simulink subsystem "station1"  (R2024b)
settings: Solver=VariableStepAuto  StartTime=0.0  StopTime=10.0  RelTol=1e-3
undefined symbols (not defined in the file): DiscIntNeverNeededParam, DPL1ph, h, Half, R3, ResistanceM, Rt4, simetran, Ts, Zm
libraries: fl_lib x215, ee_lib x97, nesl_utility x43, spsThreePhaseHarmonicFilterLib x21, simulink x7, spsThreePhaseSeriesRLCLoadLib x7, spsThreePhaseBreakerLib x7
(part 1 of 6)
settings Model: Creator=Kyle  LastModifiedBy=CD8435

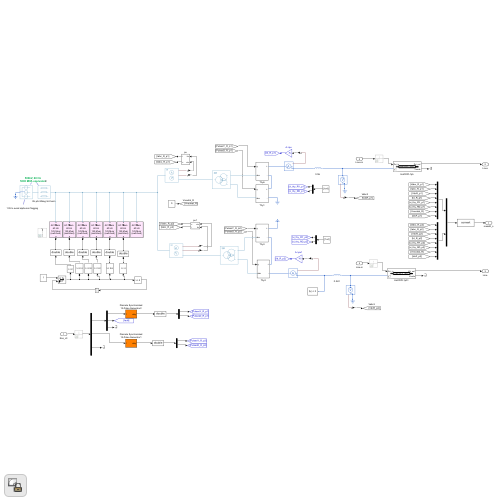
[thumbnail: Simulink's stored preview of the top-level diagram]
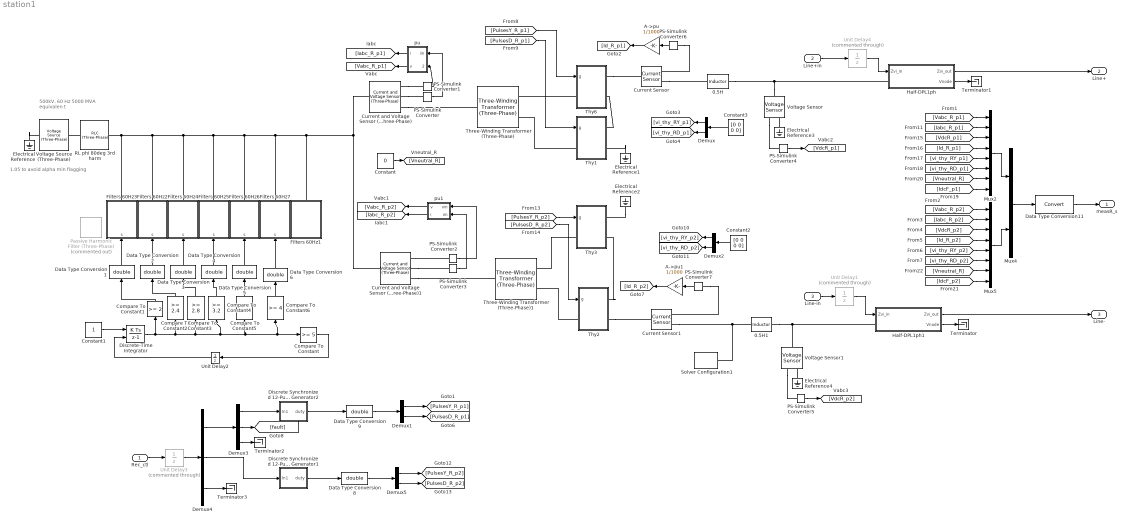
== system station1 ==
  note: 1.05 to avoid alpha min flagging
  note: 500kV, 60 Hz
      | 5000 MVA equivalen t
  Rec_ctl : Inport
  Line+in : Inport  Port=2
  Line-in : Inport  Port=3
  0.5H : ee_lib/Passive/Inductor  l=0.5 H  enable_L_tol=ee.enum.toleranceApplication.none  L_tol=20  tol_distribution=ee.enum.toleranceDistribution.uniform  nSigma=4  r=1 Ohm  g=1e-9 1/Ohm  enable_operating_limits=ee.enum.enable.no  operating_limit_action=ee.enum.passive.reportOpLim.warn  max_working_current=1 A  power_rating=1 W  fault_action=simscape.enum.assert.action.none  t_fault=1 s  i_L_specify=off  i_L_priority=High  i_L=0 A  i_L_nominal_specify=off  i_L_nominal_value=1  i_L_nominal_unit=A
  0.5H1 : ee_lib/Passive/Inductor  l=0.5 H  enable_L_tol=ee.enum.toleranceApplication.none  L_tol=20  tol_distribution=ee.enum.toleranceDistribution.uniform  nSigma=4  r=1 Ohm  g=1e-9 1/Ohm  enable_operating_limits=ee.enum.enable.no  operating_limit_action=ee.enum.passive.reportOpLim.warn  max_working_current=1 A  power_rating=1 W  fault_action=simscape.enum.assert.action.none  t_fault=1 s  i_L_specify=off  i_L_priority=High  i_L=0 A  i_L_nominal_specify=off  i_L_nominal_value=1  i_L_nominal_unit=A
  A->pu : Gain  Gain=1/1000  SaturateOnIntegerOverflow=on  OutDataTypeStr=Inherit: Same as input  ParamDataTypeStr=Inherit: Same as input
  A->pu1 : Gain  Gain=1/1000  SaturateOnIntegerOverflow=on  OutDataTypeStr=Inherit: Same as input  ParamDataTypeStr=Inherit: Same as input
  Compare To Constant : simulink/Logic and Bit Operations/Compare To Constant  relop=>=  const=5  OutDataTypeStr=uint8  ZeroCross=off
  Compare To Constant1 : simulink/Logic and Bit Operations/Compare To Constant  relop=>=  const=2  OutDataTypeStr=uint8  ZeroCross=off
  Compare To Constant2 : simulink/Logic and Bit Operations/Compare To Constant  relop=>=  const=2.4  OutDataTypeStr=uint8  ZeroCross=off
  Compare To Constant3 : simulink/Logic and Bit Operations/Compare To Constant  relop=>=  const=2.8  OutDataTypeStr=uint8  ZeroCross=off
  Compare To Constant4 : simulink/Logic and Bit Operations/Compare To Constant  relop=>=  const=3.2  OutDataTypeStr=uint8  ZeroCross=off
  Compare To Constant5 : simulink/Logic and Bit Operations/Compare To Constant  relop=>=  const=3.6  OutDataTypeStr=uint8  ZeroCross=off
  Compare To Constant6 : simulink/Logic and Bit Operations/Compare To Constant  relop=>=  const=4  OutDataTypeStr=uint8  ZeroCross=off
  Constant : Constant  Value=0
  Constant1 : Constant
  Constant2 : Constant  Value=[0 0 0 0]
  Constant3 : Constant  Value=[0 0 0 0]
  Current Sensor : fl_lib/Electrical/Electrical Sensors/Current Sensor
  Current Sensor1 : fl_lib/Electrical/Electrical Sensors/Current Sensor
  Current and Voltage Sensor (Three-Phase) : ee_lib/Sensors & Transducers/Current and Voltage Sensor (Three-Phase)  vMeasurementType=ee.enum.vmeasurement.lg  outputUnit=ee.enum.unit.si  SRated=100e6 A*V  VRated=24e3 V  I_specify=off  I_priority=None  I=[0, 0, 0] A  I_nominal_specify=off  I_nominal_value=1  I_nominal_unit=A  V_specify=off  V_priority=None  V=[0, 0, 0] V  V_nominal_specify=off  V_nominal_value=1  V_nominal_unit=V
      settings: InternalSimscapePortConfiguration="{\"Bottom\":[],\"Left\":[{\"id\":\"N1\",\"label\":\"~1\",\"type\":\"foundation.electrical.three_phase\"}],\"Right\":[{\"id\":\"V_output\",\"label\":\"V\",\"type\":\"output\"},{\"id\":\"I_output\",\"label\":\"I\",\"type\":\"output\"},{\"id\":\"N2\",\"label\":\"~2\",\"type\":\"foundation.electrical.three_phase\"}],\"Top\":[]}"
  Current and Voltage Sensor (Three-Phase)1 : ee_lib/Sensors & Transducers/Current and Voltage Sensor (Three-Phase)  vMeasurementType=ee.enum.vmeasurement.lg  outputUnit=ee.enum.unit.si  SRated=100e6 A*V  VRated=24e3 V  I_specify=off  I_priority=None  I=[0, 0, 0] A  I_nominal_specify=off  I_nominal_value=1  I_nominal_unit=A  V_specify=off  V_priority=None  V=[0, 0, 0] V  V_nominal_specify=off  V_nominal_value=1  V_nominal_unit=V
      settings: InternalSimscapePortConfiguration="{\"Bottom\":[],\"Left\":[{\"id\":\"N1\",\"label\":\"~1\",\"type\":\"foundation.electrical.three_phase\"}],\"Right\":[{\"id\":\"V_output\",\"label\":\"V\",\"type\":\"output\"},{\"id\":\"I_output\",\"label\":\"I\",\"type\":\"output\"},{\"id\":\"N2\",\"label\":\"~2\",\"type\":\"foundation.electrical.three_phase\"}],\"Top\":[]}"
  Data Type Conversion{1..6,8..9} (8 alike) : DataTypeConversion  OutDataTypeStr=double  SaturateOnIntegerOverflow=off  RndMeth=Floor
  Data Type Conversion11 : DataTypeConversion  SaturateOnIntegerOverflow=off  RndMeth=Floor
  Demux : Demux  Outputs=2
  Demux1 : Demux  Outputs=[6 6]
  Demux2 : Demux  Outputs=2
  Demux3 : Demux  Outputs=[6 1 1]
  Demux4 : Demux  Outputs=[8 6 1]
  Demux5 : Demux  Outputs=[6 6]
  Discrete Synchronized 12-Pulse Generator1 : Subsystem
  Discrete Synchronized 12-Pulse Generator2 : Subsystem
  Discrete-Time Integrator : DiscreteIntegrator  ExternalReset=rising  SampleTime=Ts  ICPrevOutput=DiscIntNeverNeededParam  ICPrevScaledInput=DiscIntNeverNeededParam
  Electrical Reference{,1..4} (5 alike) : fl_lib/Electrical/Electrical Elements/Electrical Reference
  Filters 60Hz1 : Subsystem
      mask Display: disp('AC filters \n60 Hz\n125 Mvar\n(switched)')
  Filters 60Hz2 : Subsystem
      mask Display: disp('AC filters \n60 Hz\n125 Mvar\n(switched)')
  Filters 60Hz3 : Subsystem
      mask Display: disp('AC filters \n60 Hz\n125 Mvar\n(switched)')
  Filters 60Hz4 : Subsystem
      mask Display: disp('AC filters \n60 Hz\n125 Mvar\n(switched)')
  Filters 60Hz5 : Subsystem
      mask Display: disp('AC filters \n60 Hz\n125 Mvar\n(switched)')
  Filters 60Hz6 : Subsystem
      mask Display: disp('AC filters \n60 Hz\n125 Mvar\n(switched)')
  Filters 60Hz7 : Subsystem
      mask Display: disp('AC filters \n60 Hz\n125 Mvar\n(switched)')
  Half-DPL1ph : Subsystem  AncestorBlock=simetran/Half-DPL1ph  mask(Simscape 1-phase Distributed Parameters Line){Phases=1, Frequency=60, Resistance=0.015, Inductance=0.792e-3, Capacitance=14.4e-9, Length=300, Ts=Ts, cd=on}
      mask prompts: Phases "Number of phases N"; Frequency "Frequency used for R L C specification (Hz)"; Resistance "Resistance per unit length (Ohms/km)   [N*N matrix] or [R1 R0 R0m]"; Inductance "Inductance per unit length (H/km) [N*N matrix ] or [L1 L0 L0m]"; Capacitance "Capacitance per unit length (F/km) [N*N matrix] or [C1 C0 C0m]"; Length "Line length (km)"; Ts "Sample time (s)"; cd "Compensate for explicit external Unit Delay of propagation"
      mask help:
      | Implements a single-phase distributed parameter line (DPL) model.
      |
      | This DPL model allows the decoupling of computational tasks at each line ends.
      mask init:
      | % Get current block
      | currentBlock = gcb;
      | 
      | % Get electric variables
      | [Zm,R,v,Ti,to,Rt4,h,Zimp,Zmat,Yphase,ResistanceM] = ssc_dpl_cb(gcb,'variable_mask_maskinitialization', Phases, Frequency, Resistance, Inductance, Capacitance, Length);
      | % nphase=Phases;
      | % [Zm,R,v,Ti]=powericon('Distributed Parameter Line Model',nphase,Frequency,Resistance,Inductance,Capacitance);
      | %         %[Zmxx,Rmxx,Smodexx,Tixx] = blmodlin(nphase,Frequency,Resistance,Inductance,Capacitance);
      | %         %warning(w);
      | % 
      | % 
      | %         to = Length ./ v;
      | %         Rt4 = R * Length / 4;
      | %         h = (Zm - Rt4) ./ (Zm + Rt4);
      | %         Zimp = Zm + Rt4;
      | % 
      | %         % Calculate Zmat
      | %         Zmat = zeros(nphase);
      | %         for t = 1 : nphase
      | %             Zmat(t,t) = Zimp(t);
      | %         end
      | % 
      | %         % Calculate Y phase
      | %         Yphase=Ti*inv(Zmat)*(Ti');
      | % 
      | %         % Calculate R_x_0
      | %         ResistanceM = zeros(nphase);
      | %         for t = 1 : nphase
      | %             ResistanceM(t,t) = 1/(sum(Yphase(t,1:nphase)));
      | %         end
      | % 
      | %         % Calculate R_m_n
      | %         for t = 1 : nphase
      | %             for u = t+1: nphase
      | %                 ResistanceM(t,u) = -1/(Yphase(u,t));
      | %             end
      | %         end
      | V1_init=[0 zeros(1,Phases); 0.1 zeros(1,Phases)];
      | delay=floor(to/Ts);
      | if cd==1
      |     delay=delay-1;
      | end
      | if delay<1
      |     error('Line delay is less than 1 time step');
      | end
      | remd=rem(to,Ts)/Ts;
      mask TypeOptions Phases: 1 | 2 | 3 | 4 | 5 | 6 | 8 | 9 | 10 | 12
      mask Display:
      | plot(0,0,100,100,[20,20,80,80,90,80,80,20,20,10],[50,40,40,50,50,50,61,61,50,50])
      | disp('half-DPL 1ph)')
      | %disp(mess)
  Half-DPL1ph1 : Subsystem  AncestorBlock=simetran/Half-DPL1ph  mask(Simscape 1-phase Distributed Parameters Line){Phases=1, Frequency=60, Resistance=0.015, Inductance=0.792e-3, Capacitance=14.4e-9, Length=300, Ts=Ts, cd=on}
      mask prompts: Phases "Number of phases N"; Frequency "Frequency used for R L C specification (Hz)"; Resistance "Resistance per unit length (Ohms/km)   [N*N matrix] or [R1 R0 R0m]"; Inductance "Inductance per unit length (H/km) [N*N matrix ] or [L1 L0 L0m]"; Capacitance "Capacitance per unit length (F/km) [N*N matrix] or [C1 C0 C0m]"; Length "Line length (km)"; Ts "Sample time (s)"; cd "Compensate for explicit external Unit Delay of propagation"
      mask help:
      | Implements a single-phase distributed parameter line (DPL) model.
      |
      | This DPL model allows the decoupling of computational tasks at each line ends.
      mask init: same as station1/Half-DPL1ph
      mask TypeOptions Phases: 1 | 2 | 3 | 4 | 5 | 6 | 8 | 9 | 10 | 12
      mask Display:
      | plot(0,0,100,100,[20,20,80,80,90,80,80,20,20,10],[50,40,40,50,50,50,61,61,50,50])
      | disp('half-DPL 1ph)')
      | %disp(mess)
  Mux2 : Mux  Inputs=[3 3 1 1 2 2 1 1]
  Mux4 : Mux  Inputs=[14 14 ]
  Mux5 : Mux  Inputs=[3 3 1 1 2 2 1 1]
  PS-Simulink Converter{,1..7} (8 alike) : nesl_utility/PS-Simulink Converter  PhysicalDomain=network_engine_domain  SubClassName=ps_output  LeftPortType=input  RightPortType=output  PseudoPeriodic=off  Frequencies=[]  VectorFormat=inherit  Unit=inherit  AffineConversion=off
  Passive Harmonic Filter (Three-Phase) : ee_lib/Passive/Passive Harmonic Filter (Three-Phase)  Commented=on  QRated=100e6 A*V  VRated=4160 V  FRated=60 Hz  qfactor=10  type_option=ee.enum.filtertype.BPsingle  connection_option=ee.enum.filterconnection.delta  ftuned=5 * 60 Hz  ftuned1=7 * 60 Hz  ftuned2=11 * 60 Hz  I_specify=off  I_priority=None  I=[0, 0, 0] A  I_nominal_specify=off  I_nominal_value=1  I_nominal_unit=A  V_specify=off  V_priority=None  V=[0, 0, 0] V  V_nominal_specify=off  V_nominal_value=1  V_nominal_unit=V
      settings: InternalSimscapePortConfiguration="{\"Bottom\":[],\"Left\":[{\"id\":\"N\",\"label\":\"~\",\"type\":\"foundation.electrical.three_phase\"}],\"Right\":[],\"Top\":[]}"
  RL phi 80deg 3rd harm : ee_lib/Passive/RLC Assemblies/RLC (Three-Phase)  port_option=ee.enum.threePhasePort.composite  component_structure=ee.enum.rlc.structure.ParallelRL  R=26.07 Ohm  L=48.86e-3 H  C=1e-6 F  R_parasitic=0 Ohm  G_parasitic=0 1/Ohm  IL_specify=off  IL_priority=High  IL=[0, 0, 0] A  IL_nominal_specify=off  IL_nominal_value=1  IL_nominal_unit=A  VC_specify=off  VC_priority=High  VC=[0, 0, 0] V  VC_nominal_specify=off  VC_nominal_value=1  VC_nominal_unit=V
      settings: InternalSimscapePortConfiguration="{\"Bottom\":[],\"Left\":[{\"id\":\"N1\",\"label\":\"~1\",\"type\":\"foundation.electrical.three_phase\"}],\"Right\":[{\"id\":\"N2\",\"label\":\"~2\",\"type\":\"foundation.electrical.three_phase\"}],\"Top\":[]}"
  Solver Configuration1 : nesl_utility/Solver Configuration  PhysicalDomain=network_engine_domain  SubClassName=solver  LeftPortType=input  RightPortType=generic  Tones=[]  Harmonics=[]  SimulateNoise=off  Profile=off  UseLocalSampling=off  EnableSwitchedLinearOptims=on  FrequencyDomain=off  UseCCode=off  RelTol=0.001  AbsTol=1e-06  MinStep=1e-09  ToWorkspace=off  RevertToSquareIcSolve=off  NumHomotopyIterations=100  PhasorMode=off  PhasorModeNumHarmonics=1  ConsistencySolver=NEWTON_FTOL  IndexReductionMethod=DerivativeReplacement  DoDC=off  ResidualTolerance=0.01  ConsistencyTolSource=GLOBAL  ConsistencyAbsTol=0.001  ConsistencyRelTol=0.001  ConsistencyTolFactor=0.001  UseLocalSolver=on  LocalSolverChoice=NE_BACKWARD_EULER_ADVANCER  ResolveIndetEquations=off  FunctionEvalNumThread=1  LocalSolverSampleTime=Ts  DoFixedCost=on  MaxNonlinIter=1  MaxModeIter=2  ComputeImpulses=off  ImpulseIterations=2  LinearAlgebra=Sparse  LinearAlgebraNumThread=0  EquationFormulation=NE_TIME_EF  DelaysMemoryBudget=1024  AutomaticFiltering=off  FilteringTimeConstant=0.001  PartitionStorageMethod=AS_NEEDED  PartitionMemoryBudget=1024  PartitionMethod=ROBUST  MultibodyUseLocalSolver=off  MultibodyLocalSolverChoice=ODE1  MultibodyLocalSolverSampleTime=0.001
  Terminator{,1..3} (4 alike) : Terminator
  Three-Winding Transformer (Three-Phase) : ee_lib/Passive/Transformers/Three-Winding Transformer (Three-Phase)  SRated=1200e6 A*V  FRated=60 Hz  Winding1Connection=ee.enum.windingconnection.Yg  VRated1=500e3*0.9 V  Winding2Connection=ee.enum.windingconnection.Y  VRated2=200e3 V  Winding3Connection=ee.enum.windingconnection.delta1  VRated3=200e3 V  CoreType=ee.enum.coretype.threelimb  pu_Rw1=0.0025  pu_Rw2=0.0025  pu_Rw3=0.0025  leakage_reactance_option=ee.enum.transformer_leakage.include  pu_Xl1=0.001  pu_Xl2=0.24  pu_Xl3=0.24  magnetizing_resistance_option=ee.enum.transformer_magnetizingResistance.include  pu_Rm=500  magnetizing_reactance_option=ee.enum.transformer_magnetizingReactance.exclude  saturation_option=ee.enum.transformer_saturation.exclude  pu_Xm=500  current_data=[0, .002, 1, 2]  magnetic_flux_data=[0, 1.2, 1.5, 1.51]  pu_X0=0.5  i1_specify=off  i1_priority=None  i1=[0, 0, 0] A  i1_nominal_specify=off  i1_nominal_value=1  i1_nominal_unit=A  i2_specify=off  i2_priority=None  i2=[0, 0, 0] A  i2_nominal_specify=off  i2_nominal_value=1  i2_nominal_unit=A  i3_specify=off  i3_priority=None  i3=[0, 0, 0] A  i3_nominal_specify=off  i3_nominal_value=1  i3_nominal_unit=A  phi_specify=off  phi_priority=None  phi=[0, 0, 0]  phi_nominal_specify=off  phi_nominal_value=1  phi_nominal_unit=1  power_dissipated_specify=off  power_dissipated_priority=None  power_dissipated=0 W  power_dissipated_nominal_specify=off  power_dissipated_nominal_value=1  power_dissipated_nominal_unit=W
      settings: InternalSimscapePortConfiguration="{\"Bottom\":[],\"Left\":[{\"id\":\"N1\",\"label\":\"~1\",\"type\":\"foundation.electrical.three_phase\"}],\"Right\":[{\"id\":\"N2\",\"label\":\"~2\",\"type\":\"foundation.electrical.three_phase\"},{\"id\":\"N3\",\"label\":\"~3\",\"type\":\"foundation.electrical.three_phase\"}],\"Top\":[]}"
  Three-Winding Transformer (Three-Phase)1 : ee_lib/Passive/Transformers/Three-Winding Transformer (Three-Phase)  SRated=1200e6 A*V  FRated=60 Hz  Winding1Connection=ee.enum.windingconnection.Yg  VRated1=500e3*0.9 V  Winding2Connection=ee.enum.windingconnection.Y  VRated2=200e3 V  Winding3Connection=ee.enum.windingconnection.delta1  VRated3=200e3 V  CoreType=ee.enum.coretype.fivelimb  pu_Rw1=0.0025  pu_Rw2=0.0025  pu_Rw3=0.0025  leakage_reactance_option=ee.enum.transformer_leakage.include  pu_Xl1=0.001  pu_Xl2=0.24  pu_Xl3=0.24  magnetizing_resistance_option=ee.enum.transformer_magnetizingResistance.include  pu_Rm=500  magnetizing_reactance_option=ee.enum.transformer_magnetizingReactance.exclude  saturation_option=ee.enum.transformer_saturation.exclude  pu_Xm=500  current_data=[0, .002, 1, 2]  magnetic_flux_data=[0, 1.2, 1.5, 1.51]  pu_X0=1  i1_specify=off  i1_priority=None  i1=[0, 0, 0] A  i1_nominal_specify=off  i1_nominal_value=1  i1_nominal_unit=A  i2_specify=off  i2_priority=None  i2=[0, 0, 0] A  i2_nominal_specify=off  i2_nominal_value=1  i2_nominal_unit=A  i3_specify=off  i3_priority=None  i3=[0, 0, 0] A  i3_nominal_specify=off  i3_nominal_value=1  i3_nominal_unit=A  phi_specify=off  phi_priority=None  phi=[0, 0, 0]  phi_nominal_specify=off  phi_nominal_value=1  phi_nominal_unit=1  power_dissipated_specify=off  power_dissipated_priority=None  power_dissipated=0 W  power_dissipated_nominal_specify=off  power_dissipated_nominal_value=1  power_dissipated_nominal_unit=W
      settings: InternalSimscapePortConfiguration="{\"Bottom\":[],\"Left\":[{\"id\":\"N1\",\"label\":\"~1\",\"type\":\"foundation.electrical.three_phase\"}],\"Right\":[{\"id\":\"N2\",\"label\":\"~2\",\"type\":\"foundation.electrical.three_phase\"},{\"id\":\"N3\",\"label\":\"~3\",\"type\":\"foundation.electrical.three_phase\"}],\"Top\":[]}"
  Thy1 : Subsystem
  Thy2 : Subsystem
  Thy3 : Subsystem
  Thy6 : Subsystem
  Unit Delay1 : UnitDelay  Commented=through  SampleTime=Ts  HasFrameUpgradeWarning=on
  Unit Delay2 : UnitDelay  SampleTime=Ts  HasFrameUpgradeWarning=on
  Unit Delay3 : UnitDelay  Commented=through  SampleTime=Ts  HasFrameUpgradeWarning=on
  Unit Delay4 : UnitDelay  Commented=through  SampleTime=Ts  HasFrameUpgradeWarning=on
  Voltage Source (Three-Phase) : ee_lib/Sources/Voltage Source (Three-Phase)  vline_rms=1.1*500e3 V  shift=0 deg  freq=60 Hz  impedance_option=3  SShortCircuit=1e6 A*V  XR=15  R=0.01 Ohm  L=98.03e-3 H  harmonic_option=0  harmonic_orders=[5, 7, 11, 13]  harmonic_ratios=[.1, .1, .1, .1]  G_parasitic=0 1/Ohm  I_specify=off  I_priority=None  I=[0, 0, 0] A  I_nominal_specify=off  I_nominal_value=1  I_nominal_unit=A
  Voltage Sensor : fl_lib/Electrical/Electrical Sensors/Voltage Sensor
  Voltage Sensor1 : fl_lib/Electrical/Electrical Sensors/Voltage Sensor
  pu : Subsystem  mask(PU converter){Vbase=500e3, Pbase=500e6}
      mask prompts: Vbase "Base voltage (Vrms phase-phase) :"; Pbase "Base power ( VA 3 phase)"
      mask init:
      | Kv=1/(Vbase/sqrt(3)*sqrt(2));
      | Ki=Vbase/Pbase*(sqrt(3)/sqrt(2));
  pu1 : Subsystem  mask(PU converter){Vbase=500e3, Pbase=500e6}
      mask prompts: Vbase "Base voltage (Vrms phase-phase) :"; Pbase "Base power ( VA 3 phase)"
      mask init:
      | Kv=1/(Vbase/sqrt(3)*sqrt(2));
      | Ki=Vbase/Pbase*(sqrt(3)/sqrt(2));
  measR_s : Outport
  Line+ : Outport  Port=2
  Line- : Outport  Port=3
  wires:
  Demux/1 -> [vi_thy_RY_p1]
  Demux/2 -> [vi_thy_RD_p1]
  [PulsesY_R_p1] -> Thy6/1(g)
  [PulsesD_R_p1] -> Thy1/1(g)
  Mux4/1 -> Data Type Conversion11/1
  Demux3/1 -> Discrete Synchronized 12-Pulse Generator2/1(In1)
  Demux2/1 -> [vi_thy_RY_p2]
  Demux2/2 -> [vi_thy_RD_p2]
  Rec_ctl/1 -> Unit Delay3/1
  Demux4/1 -> Demux3/1
  Demux4/2 -> Discrete Synchronized 12-Pulse Generator1/1(In1)
  [Vabc_R_p1] -> Mux2/1
  [Iabc_R_p1] -> Mux2/2
  [VdcR_p1] -> Mux2/3
  [Id_R_p1] -> Mux2/4
  [vi_thy_RY_p1] -> Mux2/5
  [vi_thy_RD_p1] -> Mux2/6
  [Vneutral_R] -> Mux2/7
  [IdcF_p1] -> Mux2/8
  [Vabc_R_p2] -> Mux5/1
  [Iabc_R_p2] -> Mux5/2
  [VdcR_p2] -> Mux5/3
  [Id_R_p2] -> Mux5/4
  [vi_thy_RY_p2] -> Mux5/5
  [vi_thy_RD_p2] -> Mux5/6
  [Vneutral_R] -> Mux5/7
  [IdcF_p2] -> Mux5/8
  Mux2/1 -> Mux4/1
  Mux5/1 -> Mux4/2
  Constant/1 -> [Vneutral_R]
  Demux4/3 -> Terminator3/1
  pu1/2(i) -> [Iabc_R_p2]
  Constant1/1 -> Discrete-Time Integrator/1
  Discrete-Time Integrator/1 -> Compare To Constant2/1, Compare To Constant/1, Compare To Constant6/1, Compare To Constant5/1, Compare To Constant4/1, Compare To Constant3/1, Compare To Constant1/1
  Compare To Constant/1 -> Unit Delay2/1
  Unit Delay2/1 -> Discrete-Time Integrator/2
  Compare To Constant1/1 -> Data Type Conversion1/1
  Compare To Constant2/1 -> Data Type Conversion2/1
  Compare To Constant3/1 -> Data Type Conversion3/1
  Compare To Constant4/1 -> Data Type Conversion4/1
  Compare To Constant5/1 -> Data Type Conversion5/1
  Compare To Constant6/1 -> Data Type Conversion6/1
  Data Type Conversion1/1 -> Filters 60Hz3/1(s)
  Data Type Conversion2/1 -> Filters 60Hz2/1(s)
  Data Type Conversion3/1 -> Filters 60Hz4/1(s)
  Data Type Conversion4/1 -> Filters 60Hz5/1(s)
  Data Type Conversion5/1 -> Filters 60Hz6/1(s)
  Data Type Conversion6/1 -> Filters 60Hz7/1(s)
  Demux1/1 -> [PulsesY_R_p1]
  Demux1/2 -> [PulsesD_R_p1]
  Demux3/2 -> [fault]
  Demux5/1 -> [PulsesY_R_p2]
  Demux5/2 -> [PulsesD_R_p2]
  Discrete Synchronized 12-Pulse Generator1/1(duty) -> Data Type Conversion8/1
  pu/2(v) -> [Vabc_R_p1]
  pu/1(i) -> [Iabc_R_p1]
  PS-Simulink Converter1/1 -> pu/2(vin)
  PS-Simulink Converter/1 -> pu/1(iin)
  PS-Simulink Converter2/1 -> pu1/1(vin)
  PS-Simulink Converter3/1 -> pu1/2(iin)
  pu1/1(v) -> [Vabc_R_p2]
  PS-Simulink Converter4/1 -> [VdcR_p1]
  PS-Simulink Converter5/1 -> [VdcR_p2]
  Data Type Conversion8/1 -> Demux5/1
  Data Type Conversion9/1 -> Demux1/1
  PS-Simulink Converter6/1 -> A->pu/1
  A->pu/1 -> [Id_R_p1]
  PS-Simulink Converter7/1 -> A->pu1/1
  [PulsesY_R_p2] -> Thy3/1(g)
  [PulsesD_R_p2] -> Thy2/1(g)
  A->pu1/1 -> [Id_R_p2]
  Constant2/1 -> Demux2/1
  Constant3/1 -> Demux/1
  Discrete Synchronized 12-Pulse Generator2/1(duty) -> Data Type Conversion9/1
  Unit Delay3/1 -> Demux4/1
  Unit Delay1/1 -> Half-DPL1ph1/1(Zvi_in)
  Unit Delay4/1 -> Half-DPL1ph/1(Zvi_in)
  Line+in/1 -> Unit Delay4/1
  Line-in/1 -> Unit Delay1/1
  Half-DPL1ph1/2(Vnode) -> Terminator/1
  Half-DPL1ph/2(Vnode) -> Terminator1/1
  Half-DPL1ph/1(Zvi_out) -> Line+/1
  Half-DPL1ph1/1(Zvi_out) -> Line-/1
  Data Type Conversion11/1 -> measR_s/1
  Demux3/3 -> Terminator2/1
  connections:
  RL phi 80deg 3rd harm/RConn1 -- Current and Voltage Sensor (Three-Phase)1/LConn1 -- Current and Voltage Sensor (Three-Phase)/LConn1 -- Filters 60Hz1/RConn1 -- Filters 60Hz7/RConn1 -- Filters 60Hz6/RConn1 -- Filters 60Hz5/RConn1 -- Filters 60Hz4/RConn1 -- Filters 60Hz2/RConn1 -- Filters 60Hz3/RConn1
  Solver Configuration1/RConn1 -- Current Sensor1/RConn2 -- 0.5H1/LConn1
  Voltage Sensor/LConn1 -- Half-DPL1ph/LConn1 -- 0.5H/RConn1
  Half-DPL1ph1/LConn1 -- Voltage Sensor1/LConn1 -- 0.5H1/RConn1
  RL phi 80deg 3rd harm/LConn1 -- Voltage Source (Three-Phase)/RConn1
  Electrical Reference/LConn1 -- Voltage Source (Three-Phase)/LConn1
  Current and Voltage Sensor (Three-Phase)/RConn2 -- PS-Simulink Converter/LConn1
  Current and Voltage Sensor (Three-Phase)/RConn1 -- PS-Simulink Converter1/LConn1
  PS-Simulink Converter2/LConn1 -- Current and Voltage Sensor (Three-Phase)1/RConn1
  Current and Voltage Sensor (Three-Phase)1/RConn2 -- PS-Simulink Converter3/LConn1
  Current Sensor/RConn2 -- 0.5H/LConn1
  Electrical Reference3/LConn1 -- Voltage Sensor/RConn2
  Voltage Sensor/RConn1 -- PS-Simulink Converter4/LConn1
  Voltage Sensor1/RConn1 -- PS-Simulink Converter5/LConn1
  Electrical Reference4/LConn1 -- Voltage Sensor1/RConn2
  Thy6/LConn1 -- Three-Winding Transformer (Three-Phase)/RConn1
  PS-Simulink Converter6/LConn1 -- Current Sensor/RConn1
  Thy1/LConn1 -- Three-Winding Transformer (Three-Phase)/RConn2
  Thy1/RConn1 -- Thy6/RConn2
  Thy6/RConn1 -- Current Sensor/LConn1
  Electrical Reference1/LConn1 -- Thy1/RConn2
  Current and Voltage Sensor (Three-Phase)/RConn3 -- Three-Winding Transformer (Three-Phase)/LConn1
  Thy2/LConn1 -- Three-Winding Transformer (Three-Phase)1/RConn2
  Thy2/RConn2 -- Current Sensor1/LConn1
  Electrical Reference2/LConn1 -- Thy3/RConn1
  Current and Voltage Sensor (Three-Phase)1/RConn3 -- Three-Winding Transformer (Three-Phase)1/LConn1
  Thy2/RConn1 -- Thy3/RConn2
  Thy3/LConn1 -- Three-Winding Transformer (Three-Phase)1/RConn1
  PS-Simulink Converter7/LConn1 -- Current Sensor1/RConn1

== system station1/Discrete Synchronized 12-Pulse Generator1 ==
  In1 : Inport
  Demux3 : Demux  Outputs=[1 1 1 1 1 1]
  Discrete Synchronized 12-Pulse Generator2 : Subsystem  mask(Discrete synchronized 12-pulse generator){pwidth=101.5, Double_Pulse=on, Ts=Ts}
      mask prompts: pwidth "Pulse width (degrees) :"; Double_Pulse "Double pulsing"; Ts "Sample time:"
      mask help:
      | Use his block  to fire the 12 thyristors of a 12-pulse converter.
      | Outputs 1 and 2 are two vectors of 6 pulses (0-1) to be sent to the two 6-pulse half bridges connected respectively to the Wye(Y) and Delta (D) connected windings of the YYD converter transformer. Pulses are individually synchronized on the 6 commutation voltages and generated alpha degrees after the increasing zero-crossings of the commutation voltages. The D pulses are lagging the Y pulses by  60 degrees.
      |
      | Input 1 is  the alpha firing signal (degrees).
      | Inputs 2, 3 and 4 are the three phase-ground synchronization voltages  measured at the  primary side of the converter transformer.
      | Input 5: Frequency of the synchronization voltages (use a constant or the Freq PLL output)
      | Input 6 allows  blocking of the pulses when the applied signal is non zero.
      |
      | When the 'Douple pulsing' option is checked, two pulses are sent to each thyristor: a 1st pulse when the aplha angle is reached, then a 2nd pulse 60 degrees later, when the next thyristor is fired.
      mask init:
      | x = [1 5; 3 5; 8 8];
      | y = [10 0; 8 2; 4 0];
      | c = [ 0.7 0.7 0.3];
  Mux1 : Mux  Inputs=2
  duty : Outport
  wires:
  In1/1 -> Demux3/1
  Demux3/1 -> Discrete Synchronized 12-Pulse Generator2/1(alpha_deg)
  Demux3/2 -> Discrete Synchronized 12-Pulse Generator2/2(A)
  Demux3/3 -> Discrete Synchronized 12-Pulse Generator2/3(B)
  Demux3/4 -> Discrete Synchronized 12-Pulse Generator2/4(C)
  Demux3/5 -> Discrete Synchronized 12-Pulse Generator2/5(Freq)
  Demux3/6 -> Discrete Synchronized 12-Pulse Generator2/6(Block)
  Discrete Synchronized 12-Pulse Generator2/1(Y) -> Mux1/1
  Discrete Synchronized 12-Pulse Generator2/2(D) -> Mux1/2
  Mux1/1 -> duty/1

== system station1/Discrete Synchronized 12-Pulse Generator2 ==
  In1 : Inport
  Demux3 : Demux  Outputs=[1 1 1 1 1 1]
  Discrete Synchronized 12-Pulse Generator2 : Subsystem  mask(Discrete synchronized 12-pulse generator){pwidth=101.5, Double_Pulse=on, Ts=Ts}
      mask prompts: pwidth "Pulse width (degrees) :"; Double_Pulse "Double pulsing"; Ts "Sample time:"
      mask help:
      | Use his block  to fire the 12 thyristors of a 12-pulse converter.
      | Outputs 1 and 2 are two vectors of 6 pulses (0-1) to be sent to the two 6-pulse half bridges connected respectively to the Wye(Y) and Delta (D) connected windings of the YYD converter transformer. Pulses are individually synchronized on the 6 commutation voltages and generated alpha degrees after the increasing zero-crossings of the commutation voltages. The D pulses are lagging the Y pulses by  60 degrees.
      |
      | Input 1 is  the alpha firing signal (degrees).
      | Inputs 2, 3 and 4 are the three phase-ground synchronization voltages  measured at the  primary side of the converter transformer.
      | Input 5: Frequency of the synchronization voltages (use a constant or the Freq PLL output)
      | Input 6 allows  blocking of the pulses when the applied signal is non zero.
      |
      | When the 'Douple pulsing' option is checked, two pulses are sent to each thyristor: a 1st pulse when the aplha angle is reached, then a 2nd pulse 60 degrees later, when the next thyristor is fired.
      mask init:
      | x = [1 5; 3 5; 8 8];
      | y = [10 0; 8 2; 4 0];
      | c = [ 0.7 0.7 0.3];
  Mux1 : Mux  Inputs=2
  duty : Outport
  wires:
  Mux1/1 -> duty/1
  Discrete Synchronized 12-Pulse Generator2/2(p D) -> Mux1/2
  Discrete Synchronized 12-Pulse Generator2/1(p Y) -> Mux1/1
  Demux3/6 -> Discrete Synchronized 12-Pulse Generator2/6(Block)
  Demux3/5 -> Discrete Synchronized 12-Pulse Generator2/5(Freq)
  Demux3/4 -> Discrete Synchronized 12-Pulse Generator2/4(C)
  Demux3/3 -> Discrete Synchronized 12-Pulse Generator2/3(B)
  Demux3/2 -> Discrete Synchronized 12-Pulse Generator2/2(A)
  Demux3/1 -> Discrete Synchronized 12-Pulse Generator2/1(alpha_deg)
  In1/1 -> Demux3/1

== system station1/Filters 60Hz1 ==
  note: Capacitor banks
  note: Tuned filters
  note: High-pass
      | damped filter
  note: 60 Hz filters 4*150 Mvars @ 500 kV
  11th 150 Mvar Q=100 : spsThreePhaseHarmonicFilterLib/Three-Phase Harmonic Filter  Commented=on  LConnTagsString=A|B|C  FilterType=Single-tuned  FilterConnection=Y (grounded)  ParNom=[500e3 60]  Qc=150e6/4  Fr=[11*60]  Frd=[11*60 13*60]  Q=100  Measurements=None
      settings: AttributesFormatString=\n
      settings: LibrarySourceBlock=|
      | sps_lib/Passives/Three-Phase
      | Harmonic Filter
  "13th 150 Mvar Q=100 " : spsThreePhaseHarmonicFilterLib/Three-Phase Harmonic Filter  Commented=on  LConnTagsString=A|B|C  FilterType=Single-tuned  FilterConnection=Y (grounded)  ParNom=[500e3 60]  Qc=150e6/4  Fr=[13*60]  Frd=[11*60 13*60]  Q=100  Measurements=None
      settings: AttributesFormatString=\n
      settings: LibrarySourceBlock=|
      | sps_lib/Passives/Three-Phase
      | Harmonic Filter
  150 Mvar : spsThreePhaseSeriesRLCLoadLib/Three-Phase Series RLC Load  Commented=on  LConnTagsString=A|B|C  Configuration=Y (grounded)  NominalVoltage=500e3  Vabc=[1e3 1e3 1e3]  Vabcp=[1e3 1e3 1e3]  NominalFrequency=60  UnbalancedPower=off  ActivePower=0  InductivePower=0  CapacitivePower=150e6/4  Pabc=[10e3 9e3 11e3]  QLabc=[100 90 110]  QCabc=[100 90 110]  Pabcp=[10e3 9e3 11e3]  QLabcp=[100 90 110]  QCabcp=[100 90 110]  Measurements=None  LoadType=constant Z
  24th 150 Mvar Q=3 : spsThreePhaseHarmonicFilterLib/Three-Phase Harmonic Filter  Commented=on  LConnTagsString=A|B|C  FilterType=High-pass  FilterConnection=Y (grounded)  ParNom=[500e3 60]  Qc=150e6/4  Fr=[24*60]  Frd=[11*60 13*60]  Q=3  Measurements=None
      settings: AttributesFormatString=\n
      settings: LibrarySourceBlock=|
      | sps_lib/Passives/Three-Phase
      | Harmonic Filter
  Electrical Reference : fl_lib/Electrical/Electrical Elements/Electrical Reference
  High-pass filter : Subsystem  mask(Three-Phase Harmonic Filter){FilterType=High-pass, FilterConnection=Y (grounded), ParNom=[500e3 60], Qc=150e6/4, Fr=[5*60], Frd=[24*60], Q=3}
      mask prompts: FilterType "Type of filter:"; FilterConnection "Filter connection:"; ParNom "Nominal L-L voltage and frequency  [Vn(Vrms) fn(Hz)]:"; Qc "Nominal reactive power (var):"; Fr "Tuning frequency (Hz)"; Frd "Tuning frequencies [ Fr1 (Hz)   Fr2 (Hz) ]"; Q "Quality factor (Q):"
      mask help:
      | Implements a three-phase harmonic filter.
      | The filter is built up from passive RLC components. Their values are computed using the specified  nominal reactive power, tuning frequency (ies) and quality factor.
      mask init:
      | [R1,L1,C1,R2,L2,C2,R3,L3,C3]=HarmonicFilterValues( FilterType, FilterConnection, ParNom, Qc, Fr, Frd, Q);
      | % Data for drawing command (Icon)
      | cx0=[0 0];
      | a=-10.5;
      | cy0=[0 a];
      | cx1=[-8 8];
      | cy1=[0 0]+a;
      | cx2=[-8 8];
      | cy2=[-5 -5]+a;
      | cx3=[0 0];
      | cy3=[a-5 a-5-11.5];
      | %
      | lx0=[0 0];
      | a=-8;
      | ly0=[0 a];
      | lx1=[0 1.4 4.3 5.7 7.1 7.7 8 7.7 7.1 5.7 4.3 1.4 0];
      | ly1=[0 0 -0.3 -0.6 -1.2 -1.5 -2.25 -3 -3.3 -3.9 -4.2 -4.5 -4.5]+a;
      | lx2=lx1;
      | ly2=ly1-4.5;
      | lx3=lx1;
      | ly3=ly1-9;
      | lx4=[0 0];
      | ly4=[a-13.5 a-13.5-5.5];
      | %
      | rx0=[0 0];
      | a=-5;
      | ry0=[0 a];
      | rx1=[0 3.8 -3.8 3.8 -3.8 3.8 -3.8 0];
      | ry1=[0 -2.5 -5 -7.5 -10 -12.5 -15 -17.5]+a;
      | rx2=[0 0];
      | ry2=[a-17.5 a-17.5-4.5];
      | %
      | switch FilterType
      | case 1,   % Single-tuned
      | 	C1_xo=50; C1_yo=85;
      | 	L1_xo=50;L1_yo=64;
      | 	R1_xo=50;R1_yo=37;
      | 	C2_xo=C1_xo;C2_yo=C1_yo;
      | 	L2_xo=L1_xo;L2_yo=L1_yo;
      |     s1x=[C2_xo C2_xo];s2x=s1x;s1y=[C2_yo C2_yo];s2y=s1y;
      |     s3x=s1x;s4x=s3x;s3y=s1y;s4y=s2y;
      | case 2,   % Double-tuned
      | 	C2_xo=78; C2_yo=40;
      | 	L2_xo=22;L2_yo=40;
      | 	C1_xo=50; C1_yo=85;
      | 	L1_xo=50;L1_yo=66;
      | 	R1_xo=50;R1_yo=40;
      |     s1x=[L2_xo C2_xo];s2x=s1x;s1y=[40 40];s2y=[13 13];
      |     s3x=s1x;s4x=s3x;s3y=s1y;s4y=s2y;
      | case 3,   % High-pass
      | 	C1_xo=50; C1_yo=75;
      | 	L1_xo=33;L1_yo=48;
      | 	R1_xo=67;R1_yo=48;
      |     C2_xo=C1_xo;C2_yo=C1_yo;
      | 	L2_xo=L1_xo;L2_yo=L1_yo;
      |     s1x=[L1_xo R1_xo];s2x=s1x;s1y=[48 48];s2y=[21 21];
      |     s3x=[C1_xo C1_xo];s4x=s3x;s3y=[21 13];s4y=[85 C1_yo];
      | case 4,   % C-type High-pass
      | 	C2_xo=33; C2_yo=58;
      | 	C1_xo=50; C1_yo=85;
      | 	L1_xo=33;L1_yo=40;
      | 	R1_xo=67;R1_yo=51;
      |     L2_xo=L1_xo;L2_yo=L1_yo;
      |     s1x=[R1_xo C2_xo];s2x=s1x;s1y=[C2_yo C2_yo];s2y=[13 13];
      |     s3x=[R1_xo R1_xo];s4x=s3x;s3y=[R1_yo C2_yo];s4y=[13 25];
      | end
      | %
      | switch FilterConnection
      | case 1,   % Y (grounded)
      |     g_xo=50;g_yo=13;
      | 	gx1=[0 0];
      |     gy1=[0 -7];
      |     gx2=[-5.5 5.5];
      |     gy2=[-7 -7];
      |     gx3=[-3 3];
      |     gy3=gy2-2;
      |     gx4=[-1.5 1.5];
      |     gy4=gy2-4;
      | case 2,   % Y (floating)
      |     g_xo=50;g_yo=13;
      | 	gx1=[0 0];
      |     gy1=[0 -10];
      |     gx2=[-4 4];
      |     gy2=[-10 -10];
      |     gx3=[-4 -4];
      |     gy3=[-7 -10];
      |     gx4=[4 4];
      |     gy4=gy3;
      | case 3,   % Y (neutral)
      | 	g_xo=50;g_yo=13;
      | 	gx1=[0 0];
      |     gy1=[0 -11];
      |     gx2=gx1;
      |     gy2=gy1;
      |     gx3=gx1;
      |     gy3=gy1;
      |     gx4=gx1;
      |     gy4=gy1;
      | case 4,   % Delta
      | 	g_xo=50;g_yo=13;
      | 	gx1=[0 0];
      |     gy1=[0 -7];
      |     gx2=[8 14];
      |     gy2=[1 1]-10;
      |     gx3=[8 11];
      |     gy3=[1 6]-10;
      |     gx4=[11 14];
      |     gy4=[6 1]-10;
      | end
      mask Help: helpview(psbhelp);
      mask TypeOptions FilterType: Single-tuned | Double-tuned | High-pass | C-type High-pass
      mask Callback FilterType: %powericon('ThreePhaseHarmonicFilterCback',gcb);
      mask TypeOptions FilterConnection: Y (grounded) | Y (floating) | Y (neutral) | Delta
      mask Callback FilterConnection: %powericon('ThreePhaseHarmonicFilterCback',gcb);
      mask Display:
      | plot(12,0,88,95)
      | plot(C1_xo+cx0,C1_yo+cy0,C1_xo+cx1,C1_yo+cy1,C1_xo+cx2,C1_yo+cy2,C1_xo+cx3,C1_yo+cy3)
      | plot(L1_xo+lx0,L1_yo+ly0,L1_xo+lx1,L1_yo+ly1,L1_xo+lx2,L1_yo+ly2,L1_xo+lx3,L1_yo+ly3,L1_xo+lx4,L1_yo+ly4)
      | plot(R1_xo+rx0,R1_yo+ry0,R1_xo+rx1,R1_yo+ry1,R1_xo+rx2,R1_yo+ry2)
      | plot(C2_xo+cx0,C2_yo+cy0,C2_xo+cx1,C2_yo+cy1,C2_xo+cx2,C2_yo+cy2,C2_xo+cx3,C2_yo+cy3)
      | plot(L2_xo+lx0,L2_yo+ly0,L2_xo+lx1,L2_yo+ly1,L2_xo+lx2,L2_yo+ly2,L2_xo+lx3,L2_yo+ly3,L2_xo+lx4,L2_yo+ly4)
      | plot(s1x,s1y,s2x,s2y,s3x,s3y,s4x,s4y)
      | plot(g_xo+gx1,g_yo+gy1,g_xo+gx2,g_yo+gy2,g_xo+gx3,g_yo+gy3,g_xo+gx4,g_yo+gy4)
  Three-Phase Breaker : spsThreePhaseBreakerLib/Three-Phase Breaker  Commented=on  InitialState=open  SwitchA=on  SwitchB=on  SwitchC=on  SwitchTimes=[1.5]  External=on  BreakerResistance=0.001  SnubberResistance=1e6  SnubberCapacitance=inf  Measurements=None
  Wye-Connected Load : ee_lib/Passive/RLC Assemblies/Wye-Connected Load  port_option=ee.enum.threePhasePort.composite  parameterization=ee.enum.rlc.parameterization.ratedpower  component_structure=ee.enum.rlc.structure.R  component_structure_PQ=ee.enum.rlc.structure.C  R=1 Ohm  L=1e-3 H  C=1e-6 F  VRated=500e3 V  FRated=60 Hz  P=1e3 W  Qpos=1e2 A*V  Qneg=-150e6/4 A*V  R_parasitic=1e-6 Ohm  G_parasitic=1e-6 1/Ohm  R_parasitic_PQ=0 Ohm  G_parasitic_PQ=1e-6 1/Ohm  Vmag0=500e3 V  Vang0=0 deg  Freq0=60 Hz  IL_specify=off  IL_priority=High  IL=[0, 0, 0] A  IL_nominal_specify=off  IL_nominal_value=1  IL_nominal_unit=A  VC_specify=off  VC_priority=High  VC=[0, 0, 0] V  VC_nominal_specify=off  VC_nominal_value=1  VC_nominal_unit=V
  tuned filter 11th : Subsystem  mask(Three-Phase Harmonic Filter){FilterType=Single-tuned, FilterConnection=Y (grounded), ParNom=[500e3 60], Qc=150e6/4, Fr=[5*60], Frd=[11*60], Q=100}
      mask prompts: FilterType "Type of filter:"; FilterConnection "Filter connection:"; ParNom "Nominal L-L voltage and frequency  [Vn(Vrms) fn(Hz)]:"; Qc "Nominal reactive power (var):"; Fr "Tuning frequency (Hz)"; Frd "Tuning frequencies [ Fr1 (Hz)   Fr2 (Hz) ]"; Q "Quality factor (Q):"
      mask help:
      | Implements a three-phase harmonic filter.
      | The filter is built up from passive RLC components. Their values are computed using the specified  nominal reactive power, tuning frequency (ies) and quality factor.
      mask init: same as station1/Filters 60Hz1/High-pass filter
      mask Help: helpview(psbhelp);
      mask TypeOptions FilterType: Single-tuned | Double-tuned | High-pass | C-type High-pass
      mask Callback FilterType: %powericon('ThreePhaseHarmonicFilterCback',gcb);
      mask TypeOptions FilterConnection: Y (grounded) | Y (floating) | Y (neutral) | Delta
      mask Callback FilterConnection: %powericon('ThreePhaseHarmonicFilterCback',gcb);
      mask Display:
      | plot(12,0,88,95)
      | plot(C1_xo+cx0,C1_yo+cy0,C1_xo+cx1,C1_yo+cy1,C1_xo+cx2,C1_yo+cy2,C1_xo+cx3,C1_yo+cy3)
      | plot(L1_xo+lx0,L1_yo+ly0,L1_xo+lx1,L1_yo+ly1,L1_xo+lx2,L1_yo+ly2,L1_xo+lx3,L1_yo+ly3,L1_xo+lx4,L1_yo+ly4)
      | plot(R1_xo+rx0,R1_yo+ry0,R1_xo+rx1,R1_yo+ry1,R1_xo+rx2,R1_yo+ry2)
      | plot(C2_xo+cx0,C2_yo+cy0,C2_xo+cx1,C2_yo+cy1,C2_xo+cx2,C2_yo+cy2,C2_xo+cx3,C2_yo+cy3)
      | plot(L2_xo+lx0,L2_yo+ly0,L2_xo+lx1,L2_yo+ly1,L2_xo+lx2,L2_yo+ly2,L2_xo+lx3,L2_yo+ly3,L2_xo+lx4,L2_yo+ly4)
      | plot(s1x,s1y,s2x,s2y,s3x,s3y,s4x,s4y)
      | plot(g_xo+gx1,g_yo+gy1,g_xo+gx2,g_yo+gy2,g_xo+gx3,g_yo+gy3,g_xo+gx4,g_yo+gy4)
  tuned filter 13th : Subsystem  mask(Three-Phase Harmonic Filter){FilterType=Single-tuned, FilterConnection=Y (grounded), ParNom=[500e3 60], Qc=150e6/4, Fr=[5*60], Frd=[13*60], Q=100}
      mask prompts: FilterType "Type of filter:"; FilterConnection "Filter connection:"; ParNom "Nominal L-L voltage and frequency  [Vn(Vrms) fn(Hz)]:"; Qc "Nominal reactive power (var):"; Fr "Tuning frequency (Hz)"; Frd "Tuning frequencies [ Fr1 (Hz)   Fr2 (Hz) ]"; Q "Quality factor (Q):"
      mask help:
      | Implements a three-phase harmonic filter.
      | The filter is built up from passive RLC components. Their values are computed using the specified  nominal reactive power, tuning frequency (ies) and quality factor.
      mask init: same as station1/Filters 60Hz1/High-pass filter
      mask Help: helpview(psbhelp);
      mask TypeOptions FilterType: Single-tuned | Double-tuned | High-pass | C-type High-pass
      mask Callback FilterType: %powericon('ThreePhaseHarmonicFilterCback',gcb);
      mask TypeOptions FilterConnection: Y (grounded) | Y (floating) | Y (neutral) | Delta
      mask Callback FilterConnection: %powericon('ThreePhaseHarmonicFilterCback',gcb);
      mask Display:
      | plot(12,0,88,95)
      | plot(C1_xo+cx0,C1_yo+cy0,C1_xo+cx1,C1_yo+cy1,C1_xo+cx2,C1_yo+cy2,C1_xo+cx3,C1_yo+cy3)
      | plot(L1_xo+lx0,L1_yo+ly0,L1_xo+lx1,L1_yo+ly1,L1_xo+lx2,L1_yo+ly2,L1_xo+lx3,L1_yo+ly3,L1_xo+lx4,L1_yo+ly4)
      | plot(R1_xo+rx0,R1_yo+ry0,R1_xo+rx1,R1_yo+ry1,R1_xo+rx2,R1_yo+ry2)
      | plot(C2_xo+cx0,C2_yo+cy0,C2_xo+cx1,C2_yo+cy1,C2_xo+cx2,C2_yo+cy2,C2_xo+cx3,C2_yo+cy3)
      | plot(L2_xo+lx0,L2_yo+ly0,L2_xo+lx1,L2_yo+ly1,L2_xo+lx2,L2_yo+ly2,L2_xo+lx3,L2_yo+ly3,L2_xo+lx4,L2_yo+ly4)
      | plot(s1x,s1y,s2x,s2y,s3x,s3y,s4x,s4y)
      | plot(g_xo+gx1,g_yo+gy1,g_xo+gx2,g_yo+gy2,g_xo+gx3,g_yo+gy3,g_xo+gx4,g_yo+gy4)
  abc : PMIOPort  Side=Right
  connections:
  abc/RConn1 -- High-pass filter/RConn1 -- tuned filter 11th/RConn1 -- Wye-Connected Load/LConn1 -- tuned filter 13th/RConn1
  Electrical Reference/LConn1 -- Wye-Connected Load/RConn1
  24th 150 Mvar Q=3/LConn3 -- "13th 150 Mvar Q=100 "/LConn3 -- 11th 150 Mvar Q=100/LConn3 -- 150 Mvar/LConn3 -- Three-Phase Breaker/LConn3
  24th 150 Mvar Q=3/LConn2 -- "13th 150 Mvar Q=100 "/LConn2 -- 11th 150 Mvar Q=100/LConn2 -- 150 Mvar/LConn2 -- Three-Phase Breaker/LConn2
  24th 150 Mvar Q=3/LConn1 -- "13th 150 Mvar Q=100 "/LConn1 -- 11th 150 Mvar Q=100/LConn1 -- 150 Mvar/LConn1 -- Three-Phase Breaker/LConn1
